simulink library "INT_EngDa_tiEngOn"  (R2016b)
settings: Solver=VariableStepAuto  StartTime=0.0  StopTime=10.0  RelTol=1e-3
settings Model: Creator=zhoutinglin  LastModifiedBy=zhoutinglin

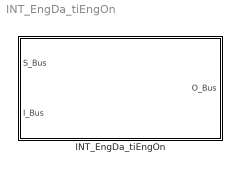
== system INT_EngDa_tiEngOn ==
  INT_EngDa_tiEngOn : Subsystem

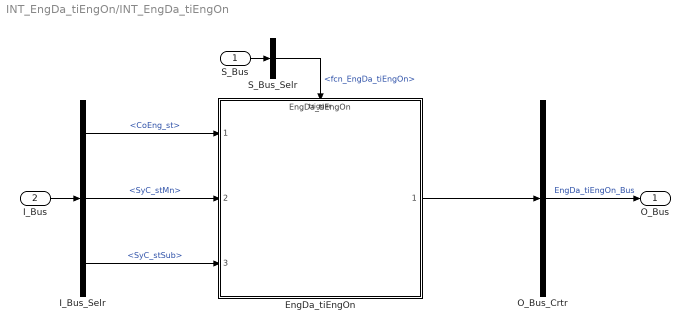
== system INT_EngDa_tiEngOn/INT_EngDa_tiEngOn ==
  S_Bus : Inport
  I_Bus : Inport  Port=2
  EngDa_tiEngOn : ModelReference  ModelNameDialog=EngDa_tiEngOn  SimulationMode=Normal  ModelReferenceVersion=1.16  TriggerPortName=function  TriggerPortTriggerType=function-call  TriggerPortStatesWhenEnabling=held
  I_Bus_Selr : BusSelector  OutputSignals=CoEng_st,SyC_stMn,SyC_stSub
  O_Bus_Crtr : BusCreator  Inputs=1
  S_Bus_Selr : BusSelector  OutputSignals=fcn_EngDa_tiEngOn
  O_Bus : Outport
  wires:
  S_Bus_Selr/1 -> EngDa_tiEngOn/Trigger  "<fcn_EngDa_tiEngOn>"
  S_Bus/1 -> S_Bus_Selr/1
  I_Bus/1 -> I_Bus_Selr/1
  I_Bus_Selr/1 -> EngDa_tiEngOn/1  "<CoEng_st>"
  I_Bus_Selr/2 -> EngDa_tiEngOn/2  "<SyC_stMn>"
  I_Bus_Selr/3 -> EngDa_tiEngOn/3  "<SyC_stSub>"
  O_Bus_Crtr/1 -> O_Bus/1  "EngDa_tiEngOn_Bus"
  EngDa_tiEngOn/1 -> O_Bus_Crtr/1
